simulink model "pole_pairs_id_Harness1"  (R2023a)
settings: configuration reference "config" (kept outside this file)
settings Model: DataDictionary=model_config.sldd  Creator=Administrator  LastModifiedBy=Administrator
settings ConfigSetRef: SourceName=config

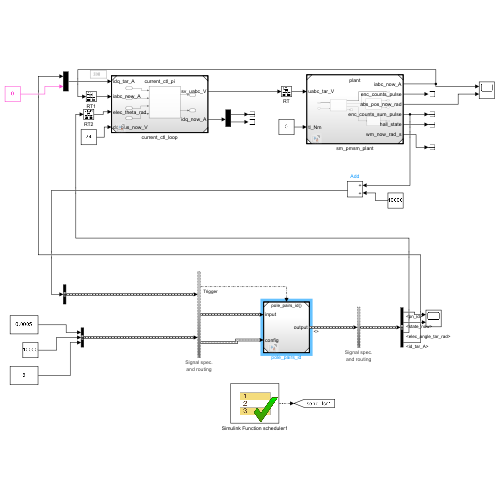
[thumbnail: Simulink's stored preview of the top-level diagram]
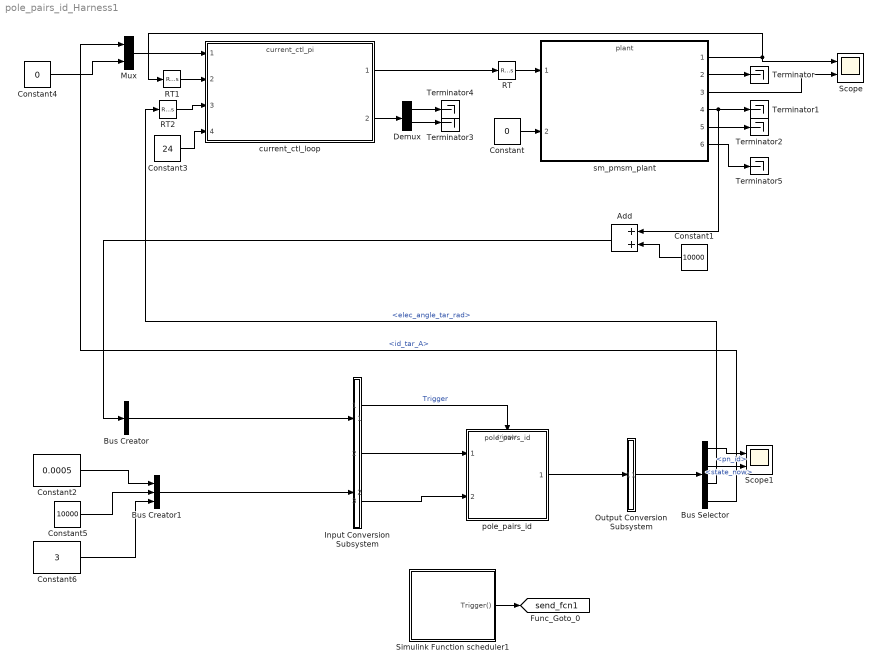
== system pole_pairs_id_Harness1 ==
  Add : Sum
  Bus Creator : BusCreator  Inputs=1  OutDataTypeStr=Bus: PolePairsIdInput  NonVirtualBus=on
      settings: InheritFromInputs=off
  Bus Creator1 : BusCreator  Inputs=3  OutDataTypeStr=Bus: PolePairsIdConfig  NonVirtualBus=on
      settings: InheritFromInputs=off
  Bus Selector : BusSelector  OutputSignals=pn_id,state_now,elec_angle_tar_rad,id_tar_A
  Constant : Constant  Value=0  OutDataTypeStr=single
  Constant1 : Constant  Value=10000  OutDataTypeStr=int64
  Constant2 : Constant  Value=0.0005  OutDataTypeStr=single
  Constant3 : Constant  Value=24  OutDataTypeStr=single
  Constant4 : Constant  Value=0  OutDataTypeStr=single
  Constant5 : Constant  Value=10000  OutDataTypeStr=uint32
  Constant6 : Constant  Value=3  OutDataTypeStr=single
  Demux : Demux  Outputs=2
  Input Conversion Subsystem : Subsystem  Tag=__SLT_ICS__  Description=|
      | Signal spec.
      | and routing
      settings: AttributesFormatString=%<Description>
  Mux : Mux  Inputs=2
  Output Conversion Subsystem : Subsystem  Tag=__SLT_OCS__  Description=|
      | Signal spec.
      | and routing
      settings: AttributesFormatString=%<Description>
  RT : RateTransition  OutPortSampleTime=1e-5
  RT1 : RateTransition  OutPortSampleTime=5e-5
  RT2 : RateTransition  OutPortSampleTime=5e-5
  Scope : Scope  NumInputPorts=2
  Scope1 : Scope  NumInputPorts=2
  Simulink Function scheduler1 : Test Sequence  Tag=__SLT_FCN_CALL__  TreatAsAtomicUnit=on
  Terminator{,1..5} (6 alike) : Terminator
  current_ctl_loop : ModelReference  ModelNameDialog=current_ctl_pi.slx  UsingDefaultArgumentValue=0,0,0,0,0,0,0,0,0  SimulationMode=Normal  ModelReferenceVersion=2.139
  pole_pairs_id : ModelReference  ModelNameDialog=pole_pairs_id  SimulationMode=Normal  ModelReferenceVersion=2.874  TriggerPortName=Trigger  TriggerPortTriggerType=function-call  TriggerPortStatesWhenEnabling=held
  sm_pmsm_plant : ModelReference  ModelNameDialog=plant.slx  UsingDefaultArgumentValue=0,0,0,0,0,0,0,0,0,0,0,0,0,0,0  SimulationMode=Normal  ModelReferenceVersion=1.26
  tag scope: send_fcn1=global
  wires:
  Bus Creator/1 -> Input Conversion Subsystem/1(Inport_1)
  Bus Creator1/1 -> Input Conversion Subsystem/2(Inport_2)
  Output Conversion Subsystem/1(Outport_1) -> Bus Selector/1
  Input Conversion Subsystem/1(Outport_3) -> pole_pairs_id/Trigger  "Trigger"
  Input Conversion Subsystem/2(Outport_1) -> pole_pairs_id/1
  Input Conversion Subsystem/3(Outport_2) -> pole_pairs_id/2
  pole_pairs_id/1 -> Output Conversion Subsystem/1(Inport_1)
  Simulink Function scheduler1/1(Trigger()) -> [send_fcn1]
  sm_pmsm_plant/4 -> Terminator1/1, Add/1
  RT/1 -> sm_pmsm_plant/1
  sm_pmsm_plant/3 -> Scope/2
  RT2/1 -> current_ctl_loop/3
  sm_pmsm_plant/2 -> Terminator/1
  Demux/1 -> Terminator4/1
  sm_pmsm_plant/5 -> Terminator2/1
  Constant3/1 -> current_ctl_loop/4
  RT1/1 -> current_ctl_loop/2
  Demux/2 -> Terminator3/1
  Constant4/1 -> Mux/2
  Constant/1 -> sm_pmsm_plant/2
  current_ctl_loop/2 -> Demux/1
  sm_pmsm_plant/1 -> Scope/1, RT1/1
  sm_pmsm_plant/6 -> Terminator5/1
  current_ctl_loop/1 -> RT/1
  Mux/1 -> current_ctl_loop/1
  Bus Selector/3 -> RT2/1  "<elec_angle_tar_rad>"
  Bus Selector/1 -> Scope1/1  "<pn_id>"
  Bus Selector/2 -> Scope1/2  "<state_now>"
  Constant2/1 -> Bus Creator1/1
  Constant5/1 -> Bus Creator1/2
  Constant6/1 -> Bus Creator1/3
  Bus Selector/4 -> Mux/1  "<id_tar_A>"
  Add/1 -> Bus Creator/1
  Constant1/1 -> Add/2

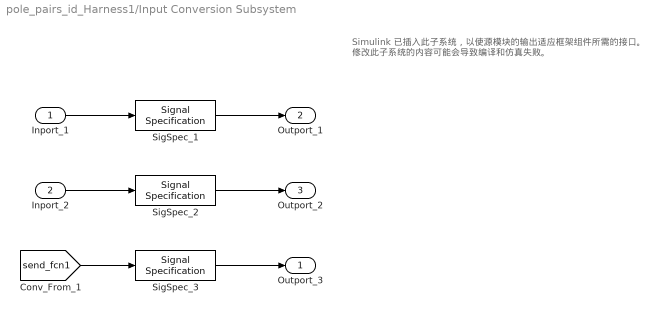
== system pole_pairs_id_Harness1/Input Conversion Subsystem ==
  note: Simulink 已插入此子系统，以使源模块的输出适应框架组件所需的接口。
      |  修改此子系统的内容可能会导致编译和仿真失败。
  Inport_1 : Inport
  Inport_2 : Inport  Port=2
  SigSpec_1 : SignalSpecification  OutDataTypeStr=Bus: PolePairsIdInput  Dimensions=[1]  BusOutputAsStruct=on
  SigSpec_2 : SignalSpecification  OutDataTypeStr=Bus: PolePairsIdConfig  Dimensions=[1]  BusOutputAsStruct=on
  SigSpec_3 : SignalSpecification
  Outport_3 : Outport
  Outport_1 : Outport  Port=2
  Outport_2 : Outport  Port=3
  wires:
  SigSpec_1/1 -> Outport_1/1
  Inport_1/1 -> SigSpec_1/1
  SigSpec_2/1 -> Outport_2/1
  Inport_2/1 -> SigSpec_2/1
  SigSpec_3/1 -> Outport_3/1
  [send_fcn1] -> SigSpec_3/1

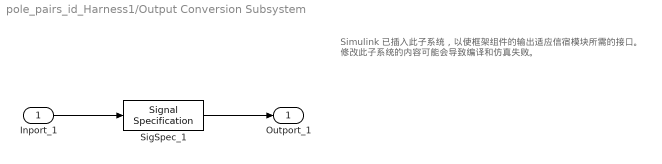
== system pole_pairs_id_Harness1/Output Conversion Subsystem ==
  note: Simulink 已插入此子系统，以使框架组件的输出适应信宿模块所需的接口。
      |  修改此子系统的内容可能会导致编译和仿真失败。
  Inport_1 : Inport
  SigSpec_1 : SignalSpecification  OutDataTypeStr=Bus: PolePairsIdOutput  Dimensions=[1]  BusOutputAsStruct=on
  Outport_1 : Outport
  wires:
  Inport_1/1 -> SigSpec_1/1
  SigSpec_1/1 -> Outport_1/1

== stateflow chart pole_pairs_id_Harness1/Simulink Function scheduler1 ==
  settings: updateMethod=DISCRETE  sampleTime=1.0E-5
  state Run
    num = 0;
    send(Trigger);
  state step_1
    num = num +1;
  state step_2
    num = 0;
    send(Trigger);
  (default) -> Run
  Run -> step_1 : [
      | true
      | ]
  step_1 -> step_2 : [
      | num >8
      | ]
  step_2 -> step_1 : [
      | true
      | ]
  data: num local
  events: Trigger output FUNCTION_CALL_EVENT
